simulink model "vs_paper2002"  (R2018a)
settings: Solver=VariableStepAuto  StartTime=0.0  StopTime=10.0  RelTol=1e-3
undefined symbols (not defined in the file): theta_0, x_0, x_ref
settings Model: Creator=hkedw  LastModifiedBy=hkedw

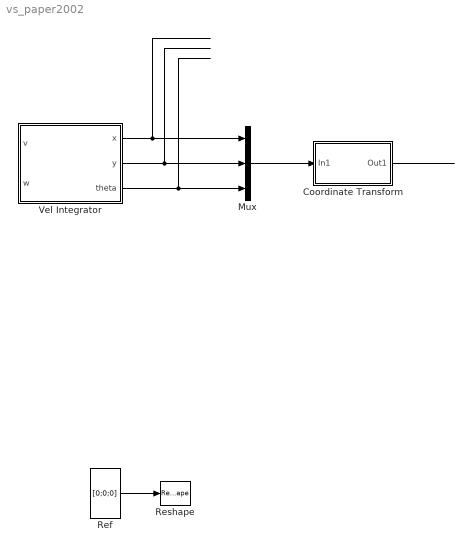
== system vs_paper2002 ==
  Coordinate Transform : Subsystem
  Mux : Mux  Inputs=3
  Ref : Constant  Value=[0;0;0]  VectorParams1D=off
  Reshape : Reshape  OutputDimensionality=Column vector (2-D)
  Vel Integrator : Subsystem
  wires:
  ? -> Vel Integrator/2(w)
  Vel Integrator/2(y) -> Mux/2
  Vel Integrator/3(theta) -> Mux/3
  Vel Integrator/1(x) -> Mux/1
  ? -> Vel Integrator/1(v)
  Ref/1 -> Reshape/1
  Mux/1 -> Coordinate Transform/1(In1)
  Coordinate Transform/1(Out1) -> ?

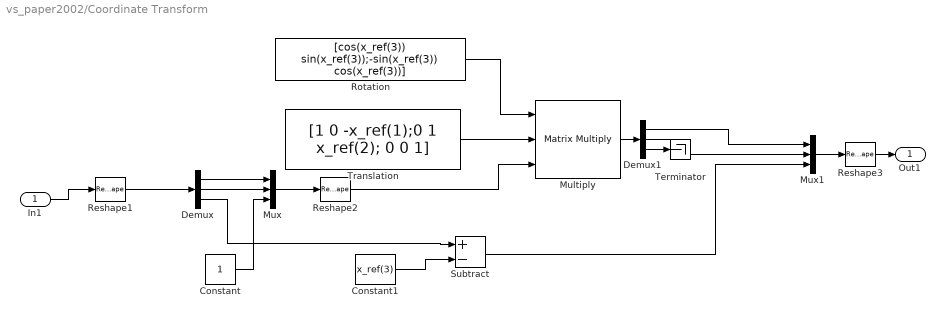
== system vs_paper2002/Coordinate Transform ==
  In1 : Inport
  Constant : Constant
  Constant1 : Constant  Value=x_ref(3)
  Demux : Demux  Outputs=3
  Demux1 : Demux  Outputs=3
  Multiply : Product  Inputs=3  Multiplication=Matrix(*)
  Mux : Mux  Inputs=3
  Mux1 : Mux  Inputs=3
  Reshape1 : Reshape  OutputDimensionality=Column vector (2-D)
  Reshape2 : Reshape  OutputDimensionality=Column vector (2-D)
  Reshape3 : Reshape  OutputDimensionality=Column vector (2-D)
  Rotation : Constant  Value=[cos(x_ref(3)) sin(x_ref(3));-sin(x_ref(3)) cos(x_ref(3))]  VectorParams1D=off
  Subtract : Sum  Inputs=+-
  Terminator : Terminator
  Translation : Constant  Value=[1 0 -x_ref(1);0 1 x_ref(2); 0 0 1]  VectorParams1D=off
  Out1 : Outport
  wires:
  Demux1/1 -> Mux1/1
  Subtract/1 -> Mux1/3
  Reshape2/1 -> Multiply/3
  Demux1/3 -> Terminator/1
  Demux/2 -> Mux/2
  Reshape1/1 -> Demux/1
  Demux/1 -> Mux/1
  Constant/1 -> Mux/3
  Demux/3 -> Subtract/1
  Demux1/2 -> Mux1/2
  Mux/1 -> Reshape2/1
  Translation/1 -> Multiply/2
  Mux1/1 -> Reshape3/1
  Rotation/1 -> Multiply/1
  Constant1/1 -> Subtract/2
  Multiply/1 -> Demux1/1
  In1/1 -> Reshape1/1
  Reshape3/1 -> Out1/1

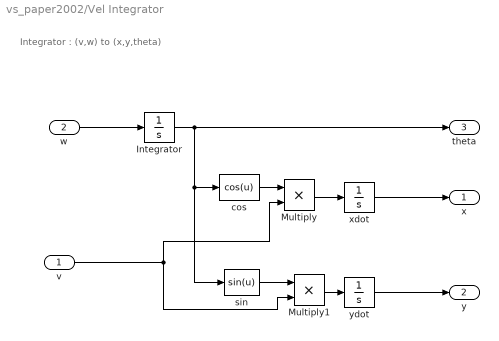
== system vs_paper2002/Vel Integrator ==
  note: Integrator : (v,w) to (x,y,theta)
  v : Inport
  w : Inport  Port=2
  Integrator : Integrator  InitialCondition=theta_0
  Multiply : Product
  Multiply1 : Product
  cos : MATLABFcn  MATLABFcn=cos(u)
  sin : MATLABFcn  MATLABFcn=sin(u)
  xdot : Integrator  InitialCondition=x_0
  ydot : Integrator  InitialCondition=x_0
  x : Outport
  y : Outport  Port=2
  theta : Outport  Port=3
  wires:
  w/1 -> Integrator/1
  Multiply/1 -> xdot/1
  cos/1 -> Multiply/1
  Multiply1/1 -> ydot/1
  ydot/1 -> y/1
  xdot/1 -> x/1
  sin/1 -> Multiply1/1
  Integrator/1 -> theta/1, sin/1, cos/1
  v/1 -> Multiply/2, Multiply1/2
